simulink subsystem "Electric_motor"  (R2023a)
settings: Solver=VariableStepAuto  StartTime=0.0  StopTime=10.0  RelTol=1e-3
undefined symbols (not defined in the file): J_engine, Km, Kw, L, R
settings Model: Creator=ycheb  LastModifiedBy=ycheb

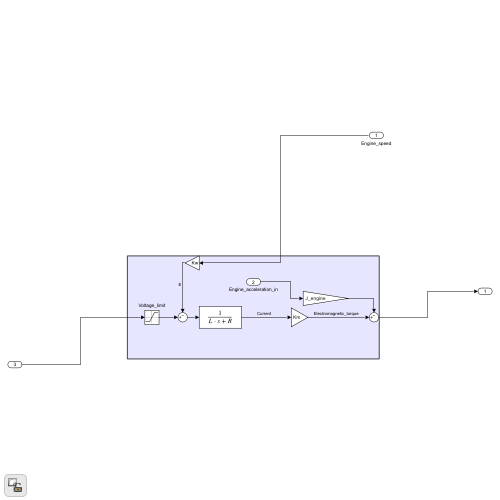
[thumbnail: Simulink's stored preview of the top-level diagram]
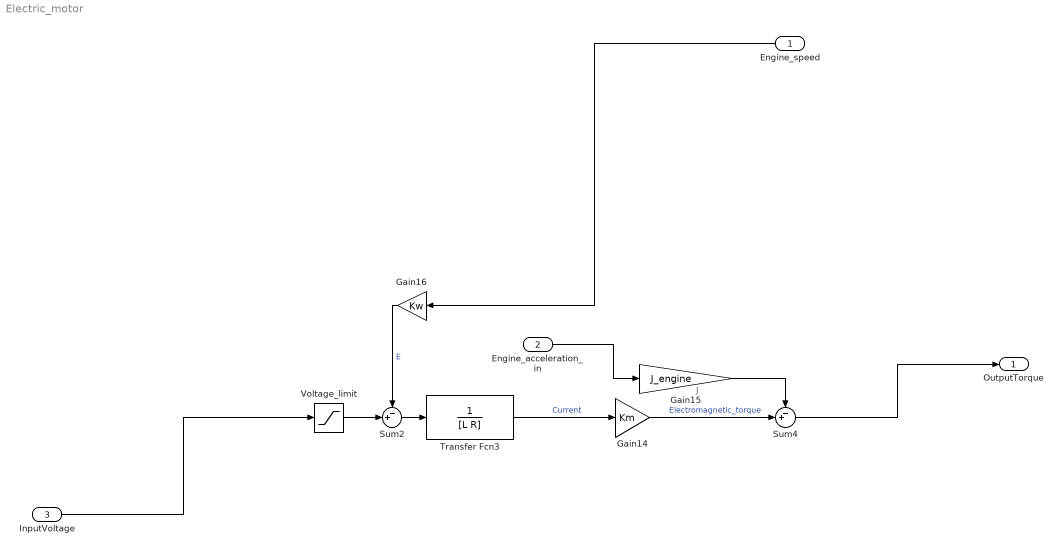
== system Electric_motor ==
  note: J
  Engine_speed : Inport
  Engine_acceleration_in : Inport  Port=2
  InputVoltage : Inport  Port=3
  Gain14 : Gain  Gain=Km
  Gain15 : Gain  Gain=J_engine
  Gain16 : Gain  Gain=Kw
  Sum2 : Sum  Inputs=-+|
  Sum4 : Sum  Inputs=-+|
  Transfer Fcn3 : TransferFcn  Denominator=[L R]
  Voltage_limit : Saturate  UpperLimit=10.8  LowerLimit=-10.8
  OutputTorque : Outport
  wires:
  Engine_speed/1 -> Gain16/1
  Sum2/1 -> Transfer Fcn3/1
  Gain15/1 -> Sum4/1
  Gain14/1 -> Sum4/2  "Electromagnetic_torque"
  Engine_acceleration_in/1 -> Gain15/1
  Transfer Fcn3/1 -> Gain14/1  "Сurrent"
  Gain16/1 -> Sum2/1  "E"
  Voltage_limit/1 -> Sum2/2
  Sum4/1 -> OutputTorque/1
  InputVoltage/1 -> Voltage_limit/1
